simulink model "NPC"  (R2015a)
settings: Solver=ode45  StartTime=0.0  StopTime=0.1  MaxStep=0.000001  MinStep=0.0000001  RelTol=1e-3
libraries: powerlib x18, simulink x1
settings Model: Creator=hp  LastModifiedBy=hp
settings SolverCC: ZeroCrossControl=DisableAll

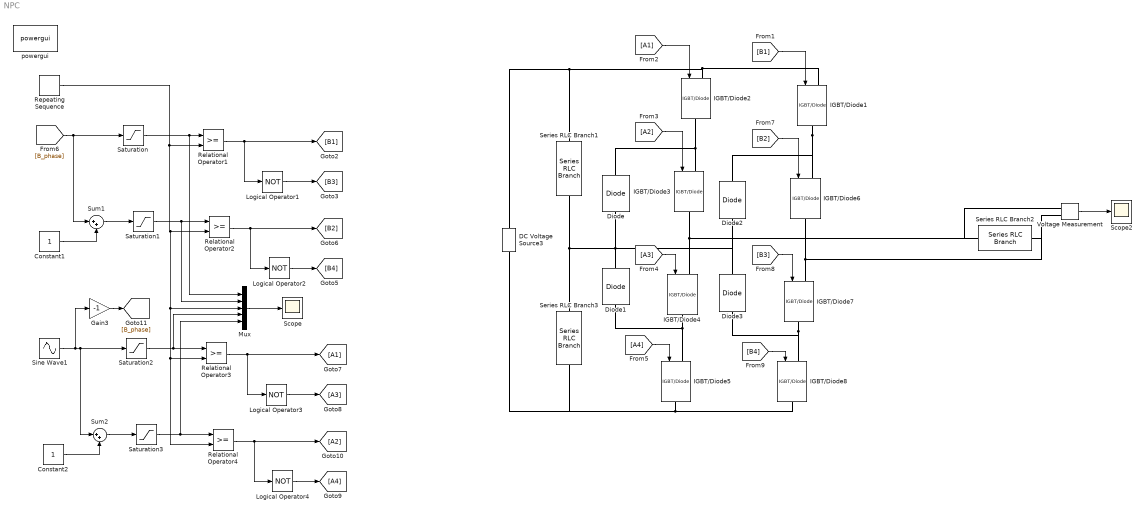
== system NPC ==
  Constant1 : Constant
  Constant2 : Constant
  DC Voltage Source3 : powerlib/Electrical Sources/DC Voltage Source  Amplitude=100  Measurements=None
  Diode{,1..3} (4 alike) : powerlib/Power Electronics/Diode  Ron=0.001  Lon=0  Vf=0.8  IC=0  UseSnubber=off  Rs=500  Cs=250e-9  Measurements=off
  Gain3 : Gain  Gain=-1
  IGBT/Diode{1..8} (8 alike) : powerlib/Power Electronics/IGBT//Diode  Ron=1e-3  Rs=1e5  Cs=inf  Measurements=off
  Logical Operator{1..4} (4 alike) : Logic  Operator=NOT  Inputs=1  AllPortsSameDT=off  OutDataTypeStr=boolean
  Mux : Mux  Inputs=5
  Relational Operator{1..4} (4 alike) : RelationalOperator  OutDataTypeStr=boolean
  Repeating Sequence : simulink/Sources/Repeating Sequence  rep_seq_t=[0 0.5 1]/1000  rep_seq_y=[0 1 0]
  Saturation{,1..3} (4 alike) : Saturate  UpperLimit=1.0  LowerLimit=0
  Scope : Scope
  Scope2 : Scope
      settings: SaveName=ScopeData2
  Series RLC Branch1 : powerlib/Elements/Series RLC Branch  LConnTagsString=__new0  RConnTagsString=__new0  BranchType=RC  Resistance=0.01  Inductance=0  SetiL0=off  InitialCurrent=0  Capacitance=4700e-5  Setx0=off  InitialVoltage=0  Measurements=None
  Series RLC Branch2 : powerlib/Elements/Series RLC Branch  LConnTagsString=__new0  RConnTagsString=__new0  BranchType=RL  Resistance=10  Inductance=0  SetiL0=off  InitialCurrent=0  Capacitance=0  Setx0=off  InitialVoltage=0  Measurements=None
  Series RLC Branch3 : powerlib/Elements/Series RLC Branch  LConnTagsString=__new0  RConnTagsString=__new0  BranchType=RC  Resistance=0.01  Inductance=0  SetiL0=off  InitialCurrent=0  Capacitance=4700e-5  Setx0=off  InitialVoltage=0  Measurements=None
  Sine Wave1 : Sin  Amplitude=0.9  Frequency=2*pi*50  SampleTime=0
  Sum1 : Sum  Inputs=|++
  Sum2 : Sum  Inputs=|++
  Voltage Measurement : powerlib/Measurements/Voltage Measurement  PhasorSimulation=off  OutputType=Complex  PSBequivalent=0
  powergui : powerlib/powergui  Priority=1  SimulationMode=Continuous  SolverType=Tustin/Backward Euler (TBE)  SampleTime=50e-6  frequency=60  SPID=off  DisableSnubberDevices=off  DisableRonSwitches=off  DisableVfSwitches=off  SwTol=0  DisplayEquations=off  Interpol=off  methode=off  Ts=100  FunctionMessages=off  echomessages=off  HookPort=off  EnableUseOfTLC=off  x0status=blocks  frequencyindice=0  Pbase=100e6  ErrMax=1e-4  Iterations=50  UnitsV=kV  UnitsW=MW  buscounter=0  RestoreLinks=warning  ResistiveCurrentMeasurement=off  Frange=[0:2:500]  Ylog=off  Xlog=on  ShowGrid=off  save=off  variable=ZData  structure=ScopeData2  ZoomFFT=off  StartTime=0.0  cycles=5  DisplayStyle=1  fundamental=50  FreqAxis=off  MaxFrequency=100000  frequencyindicesteady=1  RmsSteady=1  display=off
  wires:
  [A1] -> IGBT/Diode2/1
  [A2] -> IGBT/Diode3/1
  [A3] -> IGBT/Diode4/1
  [A4] -> IGBT/Diode5/1
  Relational Operator1/1 -> Logical Operator1/1, [B1]
  Logical Operator1/1 -> [B3]
  [B_phase] -> Sum1/1, Saturation/1
  Relational Operator2/1 -> [B2], Logical Operator2/1
  Logical Operator2/1 -> [B4]
  Saturation1/1 -> Mux/2, Relational Operator2/1
  Sum1/1 -> Saturation1/1
  Constant1/1 -> Sum1/2
  Repeating Sequence/1 -> Mux/3, Relational Operator3/2, Relational Operator4/2, Relational Operator2/2, Relational Operator1/2
  Voltage Measurement/1 -> Scope2/1
  [B1] -> IGBT/Diode1/1
  [B2] -> IGBT/Diode6/1
  [B3] -> IGBT/Diode7/1
  [B4] -> IGBT/Diode8/1
  Relational Operator3/1 -> Logical Operator3/1, [A1]
  Logical Operator3/1 -> [A3]
  Relational Operator4/1 -> [A2], Logical Operator4/1
  Logical Operator4/1 -> [A4]
  Saturation3/1 -> Mux/5, Relational Operator4/1
  Sum2/1 -> Saturation3/1
  Constant2/1 -> Sum2/2
  Saturation2/1 -> Mux/4, Relational Operator3/1
  Gain3/1 -> [B_phase]
  Sine Wave1/1 -> Sum2/1, Saturation2/1, Gain3/1
  Saturation/1 -> Mux/1, Relational Operator1/1
  Mux/1 -> Scope/1
  connections:
  Series RLC Branch1/RConn1 -- Diode3/RConn1 -- Diode2/LConn1 -- Diode1/RConn1 -- Diode/LConn1 -- Series RLC Branch3/LConn1
  DC Voltage Source3/LConn1 -- Series RLC Branch3/RConn1 -- IGBT/Diode8/RConn1 -- IGBT/Diode5/RConn1
  IGBT/Diode3/LConn1 -- Diode/RConn1 -- IGBT/Diode2/RConn1
  IGBT/Diode4/LConn1 -- Voltage Measurement/LConn1 -- Series RLC Branch2/RConn1 -- IGBT/Diode3/RConn1
  IGBT/Diode5/LConn1 -- Diode1/LConn1 -- IGBT/Diode4/RConn1
  IGBT/Diode1/RConn1 -- IGBT/Diode6/LConn1 -- Diode2/RConn1
  IGBT/Diode7/LConn1 -- Voltage Measurement/LConn2 -- Series RLC Branch2/LConn1 -- IGBT/Diode6/RConn1
  IGBT/Diode7/RConn1 -- IGBT/Diode8/LConn1 -- Diode3/LConn1
  DC Voltage Source3/RConn1 -- IGBT/Diode1/LConn1 -- IGBT/Diode2/LConn1 -- Series RLC Branch1/LConn1
